simulink model "block_diagram"  (R2023b)
settings: Solver=VariableStepAuto  StartTime=0.0  StopTime=10.0  RelTol=1e-3
libraries: simulink x1
settings Model: Creator=hzl  LastModifiedBy=hzl

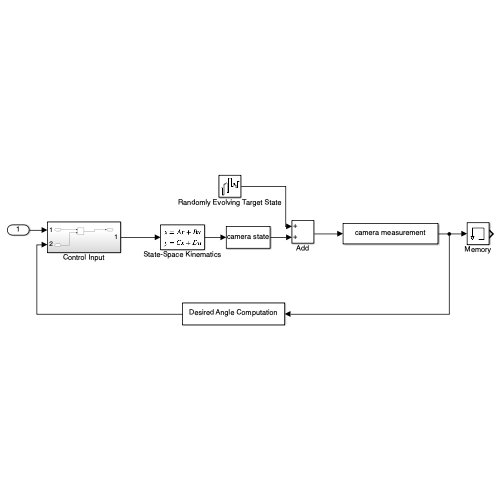
[thumbnail: Simulink's stored preview of the top-level diagram]
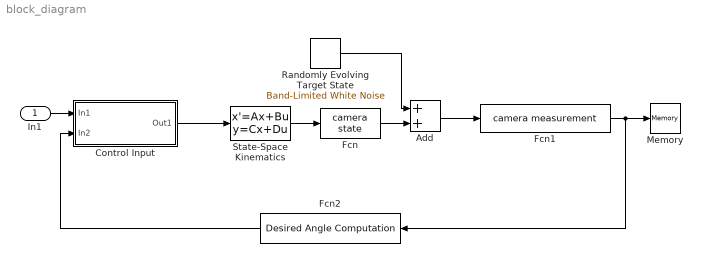
== system block_diagram ==
  In1 : Inport
  Add : Sum
  Control Input : Subsystem
  Fcn : Fcn  Expr=camera state
  Fcn1 : Fcn  Expr=camera measurement
  Fcn2 : Fcn  Expr=Desired Angle Computation
  Memory : Memory
  Randomly Evolving Target State : simulink/Sources/Band-Limited White Noise  Cov=[0.1]  Ts=0.1  seed=[23341]
  State-Space Kinematics : StateSpace  InitialCondition=0
  wires:
  Control Input/1(Out1) -> State-Space Kinematics/1
  State-Space Kinematics/1 -> Fcn/1
  Fcn1/1 -> Memory/1, Fcn2/1
  Randomly Evolving Target State/1 -> Add/1
  Fcn/1 -> Add/2
  Add/1 -> Fcn1/1
  Fcn2/1 -> Control Input/2(In2)
  In1/1 -> Control Input/1(In1)

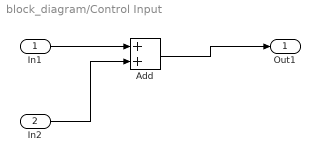
== system block_diagram/Control Input ==
  In1 : Inport
  In2 : Inport  Port=2
  Add : Sum
  Out1 : Outport
  wires:
  In1/1 -> Add/1
  Add/1 -> Out1/1
  In2/1 -> Add/2
